simulink library "gm_ZynqBF_2tx_fpga_lib"  (R2018b)
settings: Solver=VariableStepAuto  StartTime=0.0  StopTime=10.0  RelTol=1e-3
undefined symbols (not defined in the file or in its folder): Fs, ip
libraries: axiinterfacelib x4
settings Model: Creator=jason  LastModifiedBy=jason

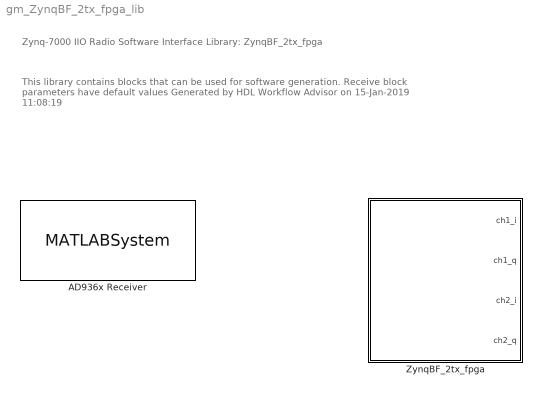
== system gm_ZynqBF_2tx_fpga_lib ==
  note: Zynq-7000 IIO Radio Software Interface Library: ZynqBF_2tx_fpga
  note: This library contains blocks that can be used for software generation.
      |
      | Receive block parameters have default values
      |
      | Generated by HDL Workflow Advisor on 15-Jan-2019 11:08:19
  AD936x Receiver : MATLABSystem  System=comm.SDRRxAD936x  IPAddress=192.168.3.2  uri=ip:10.0.0.200  CenterFrequencySource=Dialog  CenterFrequency=2.4e9  GainSource=AGC Slow Attack  Gain=10  ChannelMapping=1  BasebandSampleRate=1e6  OutputDataType=int16  SamplesPerFrame=20000  OverflowOutputPort=on  EnableBurstMode=off  NumFramesInBurst=1  ShowAdvancedProperties=off  UseCustomFilter=off  filtPathRates=[ 737280000, 11520000, 3840000, 1920000, 960000, 240000 ]  filtCoefficients=round( fir1( 127, 0.75 )*2^15*10^1.2 )  filtCoefficientSize=128  filtDecimInterpFactor=4  filtGain=-12  filtRFBandwidth=18e6  filterConfigStruct=struct()  EnableQuadratureCorrection=on  EnableRFDCCorrection=on  EnableBasebandDCCorrection=on  OverrideSampleTime=off  SampleTime=0.02  DataTimeout=Inf  ENSMPinControlMode=None  BISTLoopbackMode=Disabled  BISTToneInject=Disabled  BISTSignalGen=PRBS  BISTToneFreq=Fs/32  BISTToneLevel=0
      mask Type: comm.SDRRxAD936x
      mask Display:
      | disp(['AD936x' char(10) 'Receiver']);
      | port_label('output',1,'data');
      | port_label('output',2,'overflow');
  ZynqBF_2tx_fpga : Subsystem  TreatAsAtomicUnit=on  mask(AXI4-Lite/AXI4 Interface){}
      mask help:
      | This is an automatically generated subsystem block.
      | This contains the AXI interface blocks that communicate with the ZynqBF_2t_ip IPCore generated from ZynqBF_2tx_fpga subsystem.
      mask Display: disp(sprintf('Xilinx Zynq \nAXI Interface'));

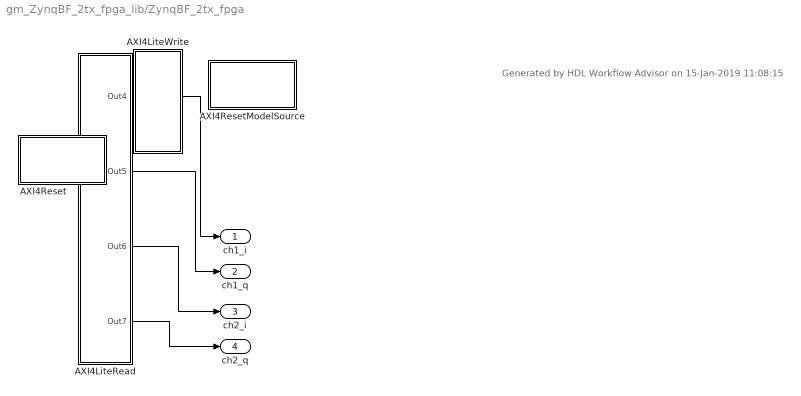
== system gm_ZynqBF_2tx_fpga_lib/ZynqBF_2tx_fpga ==
  note: Generated by HDL Workflow Advisor on 15-Jan-2019 11:08:15
  AXI4LiteRead : Subsystem  Priority=10
  AXI4LiteWrite : Subsystem  Priority=1
  AXI4Reset : Subsystem  mask(System Start){ShowInLibBrowser=0}
      mask prompts: ShowInLibBrowser "Simulink:masks:CustCodeMaskParam1_MP"
      settings: CopyFcn=cccopyfcn(gcb)  OpenFcn=ccopenfcn('System Start Function')
      mask Help: eval('feval(''rtwprivate'',''rtwhelpview'',''rtw_sys_start_block'')');
      mask Display: disp('System\nStart');
  AXI4ResetModelSource : Subsystem  mask(Model Source){ShowInLibBrowser=0}
      mask prompts: ShowInLibBrowser "Simulink:masks:CustCodeMaskParam1_MP"
      settings: CopyFcn=cccopyfcn(gcb)  OpenFcn=ccopenfcn('Model Source')
      mask Help: eval('feval(''rtwprivate'',''rtwhelpview'',''rtw_model_source_block'')');
      mask Display: disp('Model\nSource');
  ch1_i : Outport  OutDataTypeStr=fixdt(1,16,15)
  ch1_q : Outport  Port=2  OutDataTypeStr=fixdt(1,16,15)
  ch2_i : Outport  Port=3  OutDataTypeStr=fixdt(1,16,15)
  ch2_q : Outport  Port=4  OutDataTypeStr=fixdt(1,16,15)
  wires:
  AXI4LiteRead/4(Out7) -> ch2_q/1
  AXI4LiteRead/3(Out6) -> ch2_i/1
  AXI4LiteRead/2(Out5) -> ch1_q/1
  AXI4LiteRead/1(Out4) -> ch1_i/1

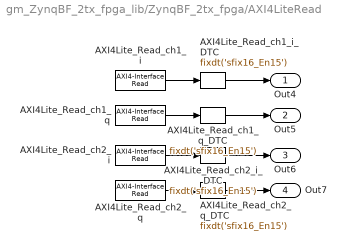
== system gm_ZynqBF_2tx_fpga_lib/ZynqBF_2tx_fpga/AXI4LiteRead ==
  AXI4Lite_Read_ch1_i : axiinterfacelib/AXI4-Interface Read  Priority=5  DeviceName=/dev/mwipcore  RegisterOffset=hex2dec('100')  DataLength=1  DataType=uint32  SampleTime=-1  blockPlatform=ZYNQ  SimulateUsing=Interpreted Execution
      settings: SourceProductName=Embedded Coder Support Package for Xilinx Zynq Platform  SourceProductBaseCode=ECZYNQ7000
  AXI4Lite_Read_ch1_i_DTC : DataTypeConversion  OutDataTypeStr=fixdt('sfix16_En15')  ConvertRealWorld=Stored Integer (SI)
  AXI4Lite_Read_ch1_q : axiinterfacelib/AXI4-Interface Read  Priority=6  DeviceName=/dev/mwipcore  RegisterOffset=hex2dec('104')  DataLength=1  DataType=uint32  SampleTime=-1  blockPlatform=ZYNQ  SimulateUsing=Interpreted Execution
      settings: SourceProductName=Embedded Coder Support Package for Xilinx Zynq Platform  SourceProductBaseCode=ECZYNQ7000
  AXI4Lite_Read_ch1_q_DTC : DataTypeConversion  OutDataTypeStr=fixdt('sfix16_En15')  ConvertRealWorld=Stored Integer (SI)
  AXI4Lite_Read_ch2_i : axiinterfacelib/AXI4-Interface Read  Priority=7  DeviceName=/dev/mwipcore  RegisterOffset=hex2dec('108')  DataLength=1  DataType=uint32  SampleTime=-1  blockPlatform=ZYNQ  SimulateUsing=Interpreted Execution
      settings: SourceProductName=Embedded Coder Support Package for Xilinx Zynq Platform  SourceProductBaseCode=ECZYNQ7000
  AXI4Lite_Read_ch2_i_DTC : DataTypeConversion  OutDataTypeStr=fixdt('sfix16_En15')  ConvertRealWorld=Stored Integer (SI)
  AXI4Lite_Read_ch2_q : axiinterfacelib/AXI4-Interface Read  Priority=8  DeviceName=/dev/mwipcore  RegisterOffset=hex2dec('10C')  DataLength=1  DataType=uint32  SampleTime=-1  blockPlatform=ZYNQ  SimulateUsing=Interpreted Execution
      settings: SourceProductName=Embedded Coder Support Package for Xilinx Zynq Platform  SourceProductBaseCode=ECZYNQ7000
  AXI4Lite_Read_ch2_q_DTC : DataTypeConversion  OutDataTypeStr=fixdt('sfix16_En15')  ConvertRealWorld=Stored Integer (SI)
  Out4 : Outport
  Out5 : Outport  Port=2
  Out6 : Outport  Port=3
  Out7 : Outport  Port=4
  wires:
  AXI4Lite_Read_ch2_i/1 -> AXI4Lite_Read_ch2_i_DTC/1
  AXI4Lite_Read_ch1_q/1 -> AXI4Lite_Read_ch1_q_DTC/1
  AXI4Lite_Read_ch1_q_DTC/1 -> Out5/1
  AXI4Lite_Read_ch2_q_DTC/1 -> Out7/1
  AXI4Lite_Read_ch1_i_DTC/1 -> Out4/1
  AXI4Lite_Read_ch2_i_DTC/1 -> Out6/1
  AXI4Lite_Read_ch2_q/1 -> AXI4Lite_Read_ch2_q_DTC/1
  AXI4Lite_Read_ch1_i/1 -> AXI4Lite_Read_ch1_i_DTC/1

== system gm_ZynqBF_2tx_fpga_lib/ZynqBF_2tx_fpga/AXI4LiteWrite ==

== system gm_ZynqBF_2tx_fpga_lib/ZynqBF_2tx_fpga/AXI4Reset ==

== system gm_ZynqBF_2tx_fpga_lib/ZynqBF_2tx_fpga/AXI4ResetModelSource ==
